simulink model "IEEE_34_node_2020a_scenarios"  (R2020a)
settings: Solver=FixedStepDiscrete  StartTime=0.0  StopTime=0.001  RelTol=1e-3
InitFcn:
  | power_34NodeTestFeeder_init;
  | %=============================
  | Vnom_ph_ph = 24900;
  | Vnom = 24900/sqrt(3);
  | Vnom1_ph_ph = 4160;
  | Vnom1 = 4160/sqrt(3);
  | Degrees_ph_ph_gen1 = 0;
  | Frequency = 60;
  | Apparent_power_gen1 = 2500e3;
  | base_current=1.5e6;
  | SW850_816=1;
  | SW818_820=1;
  | SW832_858=1;
  | SW834_842=1;
  | SW836_862=1;
  | %=============================
  | %824-828===Load1=================
  | V_824_828 = [1.008 1.016 1.012];
  | Pa_824_828 = [1e-6 1e-6 4]*1e3*1;
  | Pp_824_828 = [1e-6 1e-6 2]*1e3*1;
  | Pn_824_828 = [1e-6 1e-6 1e-6]*1;
  | 
  | %820-822===Load2=================
  | V_820_822 = 0.993;
  | Pa_820_822 = 135e3*1;
  | Pp_820_822 = 70e3*1;
  | Pn_820_822 = 1e-6*1;
  | 
  | %858-834===Load3=================
  | V_858_834 = [1.034 1.032 1.034]*sqrt(3);
  | Pa_858_834 = [4 15 13]*1e3*1;
  | Pp_858_834 = [2 8 7]*1e3*1;
  | Pn_858_834 = [1e-6 1e-6 1e-6]*1;
  | 
  | %844 B.V.c===Load4================
  | V_844 = [1.031 1.029 1.031];
  | Pa_844 = [135 135 135]*1e3*1;
  | Pp_844 = [105 105 105]*1e3*1;
  | Pn_844 = [100 100 100]*1e3*1;
  | 
  | %840======Load5=================
  | V_840 = [1.03 1.029 1.031];
  | Pa_840 = [9 9 9]*1e3*1;
  | Pp_840 = [7 7 7]*1e3*1;
  | Pn_840 = [1e-6 1e-6 1e-6]*1;
  | 
  | % For Distributed Loads==================================================
  | %802-806
  | V_802_806 = [1.047 1.048 1.048];
  | Pa_802_806 = [1e-6 30 25]*1e3;
  | Pp_802_806 = [1e-6 15 14]*1e3;
  | Pn_802_806 = [1e-6 1e-6 1e-6];
  | 
  | %808-810
  | V_808_810 = 1.014;
  | Pa_808_810 = 16e3;
  | Pp_808_810 = 8e3;
  | Pn_808_810 = 1e-6;
  | 
  | %816-824
  | ... (+107 lines)
undefined symbols (not defined in the file or in its folder): Angle, C_300, C_301, C_302, C_303, C_304, Degrees_ph, ft2km, L_300, L_301, L_302, L_303, L_304, Magnitude, ph, ph_gen1, R_300, R_301, R_302, R_303, R_304, Vnom_ph
libraries: powerlib x177
(part 2 of 2)

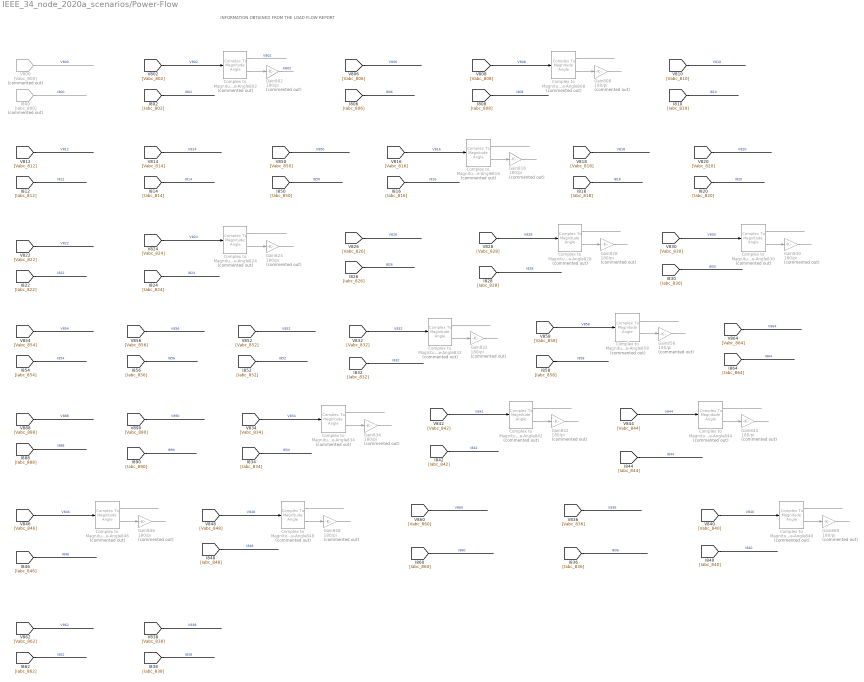
== system IEEE_34_node_2020a_scenarios/Power-Flow ==
  note: INFORMATION OBTAINED FROM THE LOAD FLOW REPORT
  Complex to Magnitude-Angle{802,808,816,824,828,830,832,834,840,842,844,846,848,858} (14 alike) : ComplexToMagnitudeAngle  Commented=on
  Gain{802,808,816,824,828,830,832,834,842,844,846,848,858,860} (14 alike) : Gain  Commented=on  Gain=180/pi
  I800 : From  Commented=on  GotoTag=Iabc_800  TagVisibility=global
  V800 : From  Commented=on  GotoTag=Vabc_800  TagVisibility=global
  wires:
  I800/1 -> ?  "I800"
  V800/1 -> ?  "V800"
  Complex to Magnitude-Angle802/2 -> Gain802/1
  Complex to Magnitude-Angle802/1 -> ?  "V802"
  [Vabc_802] -> Complex to Magnitude-Angle802/1  "V802"
  Gain802/1 -> ?  "A802"
  [Iabc_802] -> ?  "I802"
  [Vabc_806] -> ?  "V806"
  [Iabc_806] -> ?  "I806"
  Complex to Magnitude-Angle808/1 -> ?
  Complex to Magnitude-Angle808/2 -> Gain808/1
  [Iabc_808] -> ?  "I808"
  [Vabc_808] -> Complex to Magnitude-Angle808/1  "V808"
  Gain808/1 -> ?
  [Vabc_810] -> ?  "V810"
  [Iabc_810] -> ?  "I810"
  [Vabc_812] -> ?  "V812"
  [Iabc_812] -> ?  "I812"
  [Vabc_814] -> ?  "V814"
  [Iabc_814] -> ?  "I814"
  [Vabc_850] -> ?  "V850"
  [Iabc_850] -> ?  "I850"
  [Iabc_816] -> ?  "I816"
  Gain816/1 -> ?
  [Vabc_816] -> Complex to Magnitude-Angle816/1  "V816"
  Complex to Magnitude-Angle816/2 -> Gain816/1
  Complex to Magnitude-Angle816/1 -> ?
  [Vabc_818] -> ?  "V818"
  [Iabc_818] -> ?  "I818"
  [Vabc_820] -> ?  "V820"
  [Iabc_820] -> ?  "I820"
  [Vabc_822] -> ?  "V822"
  [Iabc_822] -> ?  "I822"
  Complex to Magnitude-Angle824/1 -> ?
  Gain824/1 -> ?
  [Iabc_824] -> ?  "I824"
  [Vabc_824] -> Complex to Magnitude-Angle824/1  "V824"
  Complex to Magnitude-Angle824/2 -> Gain824/1
  [Vabc_826] -> ?  "V826"
  [Iabc_826] -> ?  "I826"
  Gain828/1 -> ?
  Complex to Magnitude-Angle828/2 -> Gain828/1
  [Iabc_828] -> ?  "I828"
  Complex to Magnitude-Angle828/1 -> ?
  [Vabc_828] -> Complex to Magnitude-Angle828/1  "V828"
  Complex to Magnitude-Angle830/1 -> ?
  Gain830/1 -> ?
  Complex to Magnitude-Angle830/2 -> Gain830/1
  [Iabc_830] -> ?  "I830"
  [Vabc_830] -> Complex to Magnitude-Angle830/1  "V830"
  [Vabc_854] -> ?  "V854"
  [Iabc_854] -> ?  "I854"
  [Vabc_856] -> ?  "V856"
  [Iabc_856] -> ?  "I856"
  [Vabc_852] -> ?  "V852"
  [Iabc_852] -> ?  "I852"
  Complex to Magnitude-Angle832/1 -> ?
  [Vabc_832] -> Complex to Magnitude-Angle832/1  "V832"
  Complex to Magnitude-Angle832/2 -> Gain832/1
  Gain832/1 -> ?
  [Iabc_832] -> ?  "I832"
  [Iabc_858] -> ?  "I858"
  Complex to Magnitude-Angle858/2 -> Gain858/1
  Complex to Magnitude-Angle858/1 -> ?
  Gain858/1 -> ?
  [Vabc_858] -> Complex to Magnitude-Angle858/1  "V858"
  [Vabc_864] -> ?  "V864"
  [Iabc_864] -> ?  "I864"
  [Iabc_888] -> ?  "I888"
  [Vabc_888] -> ?  "V888"
  [Vabc_890] -> ?  "V890"
  [Iabc_890] -> ?  "I890"
  Gain834/1 -> ?
  Complex to Magnitude-Angle834/2 -> Gain834/1
  [Vabc_834] -> Complex to Magnitude-Angle834/1  "V834"
  [Iabc_834] -> ?  "I834"
  Complex to Magnitude-Angle834/1 -> ?
  Complex to Magnitude-Angle846/1 -> ?
  [Iabc_844] -> ?  "I844"
  Gain860/1 -> ?
  [Vabc_836] -> ?  "V836"
  Gain844/1 -> ?
  Complex to Magnitude-Angle840/1 -> ?
  [Vabc_860] -> ?  "V860"
  Gain846/1 -> ?
  [Iabc_840] -> ?  "I840"
  [Iabc_836] -> ?  "I836"
  Gain848/1 -> ?
  Complex to Magnitude-Angle844/2 -> Gain844/1
  [Vabc_840] -> Complex to Magnitude-Angle840/1  "V840"
  [Vabc_846] -> Complex to Magnitude-Angle846/1  "V846"
  [Iabc_848] -> ?  "I848"
  Complex to Magnitude-Angle848/2 -> Gain848/1
  Complex to Magnitude-Angle840/2 -> Gain860/1
  [Iabc_846] -> ?  "I846"
  Complex to Magnitude-Angle844/1 -> ?
  Complex to Magnitude-Angle846/2 -> Gain846/1
  [Vabc_848] -> Complex to Magnitude-Angle848/1  "V848"
  Complex to Magnitude-Angle848/1 -> ?
  [Vabc_844] -> Complex to Magnitude-Angle844/1  "V844"
  [Iabc_860] -> ?  "I860"
  [Iabc_842] -> ?  "I842"
  Gain842/1 -> ?
  Complex to Magnitude-Angle842/1 -> ?
  Complex to Magnitude-Angle842/2 -> Gain842/1
  [Vabc_842] -> Complex to Magnitude-Angle842/1  "V842"
  [Vabc_862] -> ?  "V862"
  [Iabc_862] -> ?  "I862"
  [Vabc_838] -> ?  "V838"
  [Iabc_838] -> ?  "I838"
